simulink model "cubesat_alg_dev_env_v2_demoable"  (R2023a)
settings: Solver=FixedStepAuto  StartTime=0.0  StopTime=7200  FixedStep=0.01  MaxStep=1  MinStep=0.001  RelTol=1e-3
undefined symbols (not defined in the file or in its folder): WMM2020
libraries: aerolibutil x7, matrix_library x4, sharedtransform x2, dspinverses x1, sharedutil x1, simulink_extras x1, vrlib x1, aerolibgravity2 x1
settings Model: Creator=samuel  LastModifiedBy=samuel
settings OptimizationCC: ReuseModelBlockBuffer=off
settings ModelReferenceCC: EnableRefExpFcnMdlSchedulingChecks=on

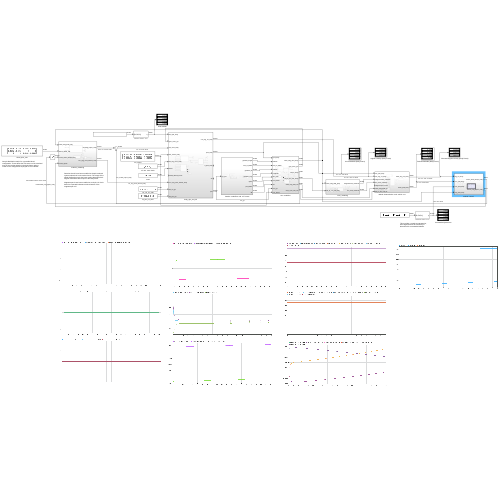
[thumbnail: Simulink's stored preview of the top-level diagram]
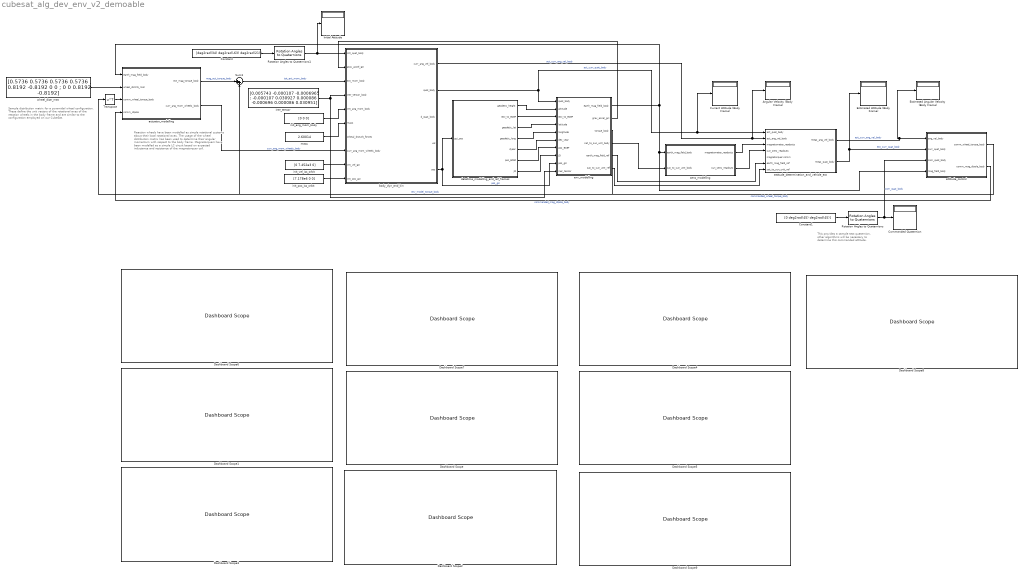
== system cubesat_alg_dev_env_v2_demoable ==
  note: This provides a sample test quaternion, other algorithms will be necessary to determine this commanded attitude.
  note: Reaction wheels have been modelled as simple rotational systems about their local rotational axes. The usage of the wheel distribution matrix has been used to determine their angular momentum with respect to the body frame.
      |
      | Magnetorquers have been modelled as a simple LC circuit based on expected inductance and resistance of the magnetorquer coil.
  note: Sample distribution matrix for a pyramidal wheel configuration. These define the unit vectors of the rotational axes of the reaction wheels in the body frame and are similar to the configuration employed on our CubeSat.
  Angular Velocity (Body Frame) : Display
  Commanded Quaternion : Display
  Constant : Constant  Value=[deg2rad(34) deg2rad(-63) deg2rad(21)]
  Constant1 : Constant  Value=[0 deg2rad(45) deg2rad(45)]
  Current Attitude (Body Frame) : Display
  Dashboard Scope{,1..9} (10 alike) : DashboardScope
  Estimated Angular Velocity (Body Frame) : Display
  Estimated Attitude (Body Frame) : Display
  Initial Attitude : Display
  Rotation Angles to Quaternions : sharedtransform/Rotation Angles to Quaternions  rotationOrder=ZYX  aMode=aMode
  Rotation Angles to Quaternions1 : sharedtransform/Rotation Angles to Quaternions  rotationOrder=ZYX  aMode=aMode
  Sum3 : Sum  Inputs=|++
  Transpose : Math  Operator=transpose
  actuator_modelling : Subsystem
  attitude_control : Subsystem
  attitude_determination_and_vehicle_est : Subsystem
  body_dyn_and_kin : Subsystem
  datetime_modelling_and_ref_frames : Subsystem
  env_modelling : Subsystem
  iner_tensor : Constant  Value=[0.005743 -0.000107 -0.0006965 ; -0.000107 0.030927 0.000086 ; -0.000696 0.000086 0.030951]
  init_ang_mom_body : Constant  Value=[0 0 0]
  init_pos_iss_orbit : Constant  Value=[7.178e6 0 0]
  init_vel_iss_orbit : Constant  Value=[0 7.452e3 0]
  mass : Constant  Value=2.60014
  sens_modelling : Subsystem
  wheel_distr_mat : Constant  Value=[0.5736 0.5736 0.5736 0.5736 ; 0.8192 -0.8192 0 0 ; 0 0 0.8192 -0.8192]
  wires:
  iner_tensor/1 -> env_modelling/10(iner_tensor), body_dyn_and_kin/4(iner_tensor_body)
  wheel_distr_mat/1 -> actuator_modelling/2(wheel_distrib_mat)
  actuator_modelling/1(ext_mag_torque_body) -> Sum3/1  "mag_act_torque_body"
  body_dyn_and_kin/2(quat_body) -> attitude_determination_and_vehicle_est/1(act_quat_body), Current Attitude (Body Frame)/1, env_modelling/1(quat_body)  "act_curr_quat_body"
  body_dyn_and_kin/5(pos) -> env_modelling/9(pos_gci), datetime_modelling_and_ref_frames/1(gci_pos)  "pos_gci"
  Sum3/1 -> body_dyn_and_kin/3(ext_mom_body)  "tot_ext_mom_body"
  init_ang_mom_body/1 -> body_dyn_and_kin/5(init_ang_mom_body)
  mass/1 -> body_dyn_and_kin/6(mass)
  actuator_modelling/2(curr_ang_mom_wheels_body) -> body_dyn_and_kin/8(curr_ang_mom_wheels_body)  "curr_ang_mom_wheels_body"
  init_vel_iss_orbit/1 -> body_dyn_and_kin/9(init_vel_gci)
  init_pos_iss_orbit/1 -> body_dyn_and_kin/10(init_pos_gci)
  env_modelling/1(earth_mag_field_body) -> attitude_control/4(mag_field_body), sens_modelling/1(earth_mag_field_body), actuator_modelling/1(earth_mag_field_body)
  datetime_modelling_and_ref_frames/1(geodetic_height) -> env_modelling/2(altitude)
  datetime_modelling_and_ref_frames/2(GCI_to_ECEF) -> env_modelling/3(GCI_to_ECEF)
  datetime_modelling_and_ref_frames/3(geodetic_lat) -> env_modelling/4(latitude)
  datetime_modelling_and_ref_frames/4(geodetic_long) -> env_modelling/5(longitude)
  datetime_modelling_and_ref_frames/5(dyear) -> env_modelling/6(dec_year)
  datetime_modelling_and_ref_frames/6(pos_ECEF) -> env_modelling/7(pos_ECEF)
  datetime_modelling_and_ref_frames/7(JD) -> env_modelling/8(JD)
  env_modelling/2(grav_accel_gci) -> body_dyn_and_kin/2(grav_accel_gci)
  env_modelling/3(torque_body) -> Sum3/2  "env_model_torque_body"
  env_modelling/4(sat_to_sun_unit_body) -> sens_modelling/2(sat_to_sun_unit_body)
  attitude_determination_and_vehicle_est/1(meas_ang_vel_body) -> Estimated Angular Velocity (Body Frame)/1, attitude_control/1(ang_vel_body)  "est_curr_ang_vel_body"
  attitude_determination_and_vehicle_est/2(meas_quat_body) -> Estimated Attitude (Body Frame)/1, attitude_control/2(curr_quat_body)  "est_curr_quat_body"
  attitude_control/1(comm_wheel_torque_body) -> Transpose/1  "commanded_wheel_torque_body"
  body_dyn_and_kin/1(curr_ang_vel_body) -> Angular Velocity (Body Frame)/1, attitude_determination_and_vehicle_est/2(act_ang_vel_body)  "act_curr_ang_vel_body"
  sens_modelling/1(magnetometer_readouts) -> attitude_determination_and_vehicle_est/3(magnetometer_readouts)
  sens_modelling/2(sun_sens_readouts) -> attitude_determination_and_vehicle_est/4(sun_sens_readouts)
  env_modelling/5(earth_mag_field_ref) -> attitude_determination_and_vehicle_est/6(earth_mag_field_ref)
  env_modelling/6(sat_to_sun_unit_ref) -> attitude_determination_and_vehicle_est/7(sat_to_sun_unit_ref)
  Transpose/1 -> actuator_modelling/3(comm_wheel_torque_body)
  Constant1/1 -> Rotation Angles to Quaternions/1
  Rotation Angles to Quaternions/1 -> Commanded Quaternion/1, attitude_control/3(com_quat_body)  "com_quat_body"
  Rotation Angles to Quaternions1/1 -> body_dyn_and_kin/1(init_quat_body), Initial Attitude/1
  Constant/1 -> Rotation Angles to Quaternions1/1
  attitude_control/2(comm_mag_dipole_body) -> actuator_modelling/4(comm_dipole)  "commanded_mag_dipole_body"

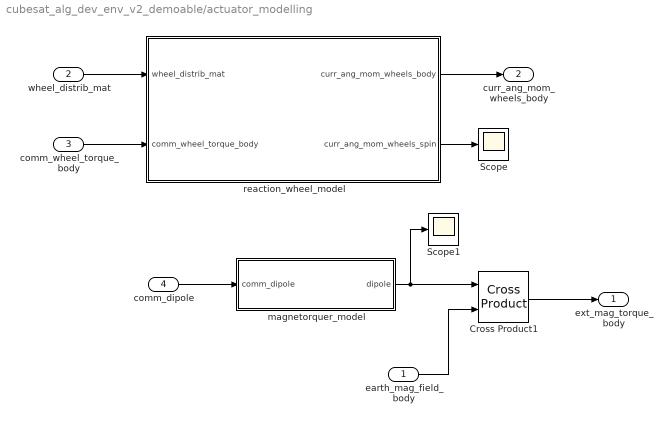
== system cubesat_alg_dev_env_v2_demoable/actuator_modelling ==
  earth_mag_field_body : Inport
  wheel_distrib_mat : Inport  Port=2
  comm_wheel_torque_body : Inport  Port=3
  comm_dipole : Inport  Port=4
  Cross Product1 : matrix_library/Cross Product
  Scope : Scope
  Scope1 : Scope
  magnetorquer_model : Subsystem
  reaction_wheel_model : Subsystem
  ext_mag_torque_body : Outport
  curr_ang_mom_wheels_body : Outport  Port=2
  wires:
  reaction_wheel_model/2(curr_ang_mom_wheels_spin) -> Scope/1
  magnetorquer_model/1(dipole) -> Scope1/1, Cross Product1/1
  Cross Product1/1 -> ext_mag_torque_body/1
  wheel_distrib_mat/1 -> reaction_wheel_model/1(wheel_distrib_mat)
  comm_wheel_torque_body/1 -> reaction_wheel_model/2(comm_wheel_torque_body)
  earth_mag_field_body/1 -> Cross Product1/2
  comm_dipole/1 -> magnetorquer_model/1(comm_dipole)
  reaction_wheel_model/1(curr_ang_mom_wheels_body) -> curr_ang_mom_wheels_body/1

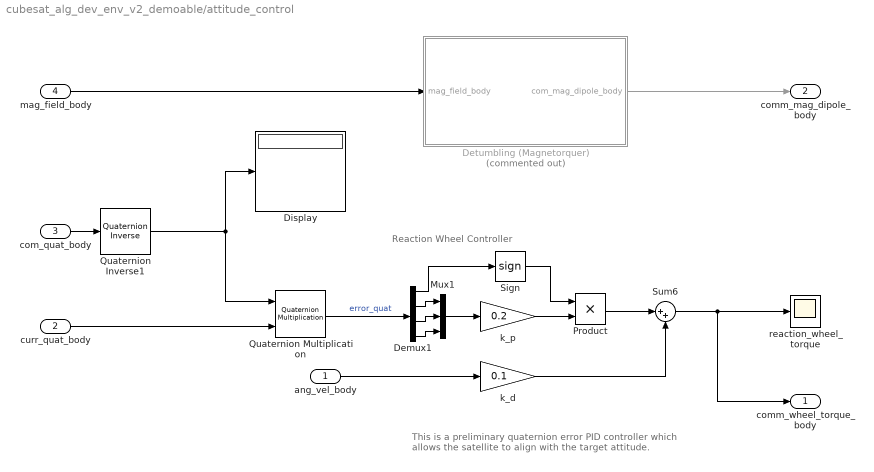
== system cubesat_alg_dev_env_v2_demoable/attitude_control ==
  note: This is a preliminary quaternion error PID controller which allows the satellite to align with the target attitude.
  note: Reaction Wheel Controller
  ang_vel_body : Inport
  curr_quat_body : Inport  Port=2
  com_quat_body : Inport  Port=3
  mag_field_body : Inport  Port=4
  Demux1 : Demux
  Detumbling (Magnetorquer) : Subsystem  Commented=on
  Display : Display
  Mux1 : Mux  Inputs=3
  Product : Product
  Quaternion Inverse1 : aerolibutil/Quaternion Inverse
  Quaternion Multiplication : aerolibutil/Quaternion Multiplication
  Sign : Signum
  Sum6 : Sum  Inputs=|++
  k_d : Gain  Gain=0.1
  k_p : Gain  Gain=0.2
  reaction_wheel_torque : Scope
  comm_wheel_torque_body : Outport
  comm_mag_dipole_body : Outport  Port=2
  wires:
  Quaternion Multiplication/1 -> Demux1/1  "error_quat"
  curr_quat_body/1 -> Quaternion Multiplication/2
  ang_vel_body/1 -> k_d/1
  Quaternion Inverse1/1 -> Display/1, Quaternion Multiplication/1
  Sum6/1 -> comm_wheel_torque_body/1, reaction_wheel_torque/1
  Demux1/3 -> Mux1/2
  Demux1/2 -> Mux1/1
  Demux1/4 -> Mux1/3
  k_p/1 -> Product/2
  Demux1/1 -> Sign/1
  Mux1/1 -> k_p/1
  Sign/1 -> Product/1
  Product/1 -> Sum6/1
  k_d/1 -> Sum6/2
  com_quat_body/1 -> Quaternion Inverse1/1
  mag_field_body/1 -> Detumbling (Magnetorquer)/1(mag_field_body)
  Detumbling (Magnetorquer)/1(com_mag_dipole_body) -> comm_mag_dipole_body/1

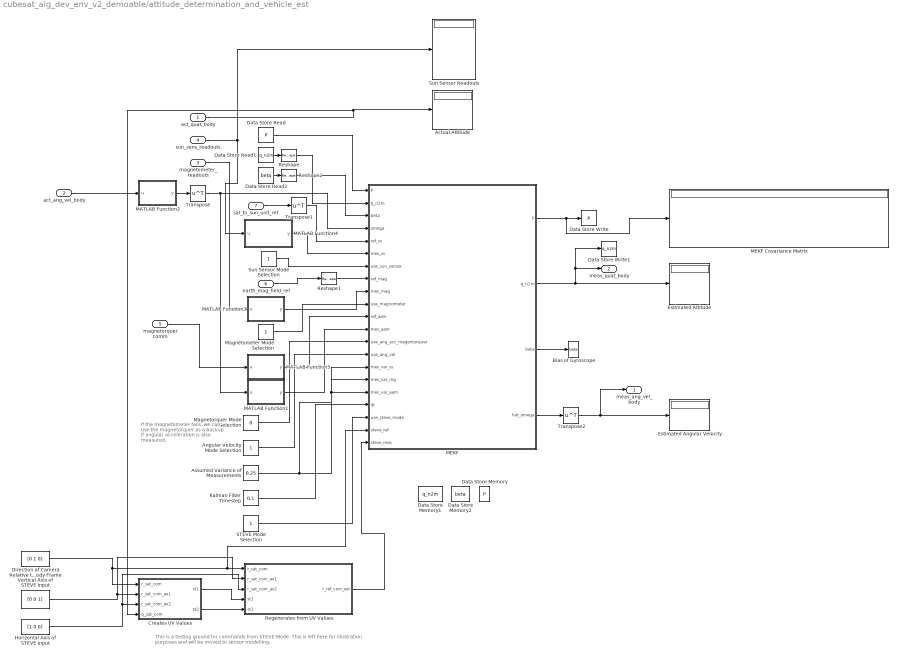
== system cubesat_alg_dev_env_v2_demoable/attitude_determination_and_vehicle_est ==
  note: This is a testing ground for commands from STEVE Mode. This is left here for illustration purposes and will be moved to sensor modelling.
  note: If the magnetometer fails, we can use the magnetorquer as a backup if angular acceleration is also measured.
  act_quat_body : Inport
  act_ang_vel_body : Inport  Port=2
  magnetometer_readouts : Inport  Port=3
  sun_sens_readouts : Inport  Port=4
  magnetorquer comm : Inport  Port=5
  earth_mag_field_ref : Inport  Port=6
  sat_to_sun_unit_ref : Inport  Port=7
  Actual Attitude : Display
  Angular Velocity Mode Selection : Constant
  Assumed Variance of Measurements : Constant  Value=0.25
  Bias of Gyroscope : DataStoreWrite  DataStoreName=beta  IndexOptions=Index vector (dialog)  Indices=1  OutputSizes=1
  Creates UV Values : MATLAB Function  TreatAsAtomicUnit=on
  Data Store Memory : DataStoreMemory  DataStoreName=P  WriteAfterWriteMsg=warning  InitialValue=diag([1*ones(1,3), 1*ones(1,3)])  ShowAdditionalParam=off
  Data Store Memory1 : DataStoreMemory  DataStoreName=q_n2m  WriteAfterWriteMsg=warning  InitialValue=[1, 0, 0, 0]  ShowAdditionalParam=off  Dimensions=[1,4]
  Data Store Memory2 : DataStoreMemory  DataStoreName=beta  WriteAfterWriteMsg=warning  InitialValue=[0;0;0]  ShowAdditionalParam=off  Dimensions=[3,1]
  Data Store Read : DataStoreRead  DataStoreName=P  IndexOptions=Index vector (dialog)  Indices=1  OutputSizes=1
  Data Store Read1 : DataStoreRead  DataStoreName=q_n2m  IndexOptions=Index vector (dialog)  Indices=1  OutputSizes=1
  Data Store Read2 : DataStoreRead  DataStoreName=beta  IndexOptions=Index vector (dialog)  Indices=1  OutputSizes=1
  Data Store Write : DataStoreWrite  DataStoreName=P  IndexOptions=Index vector (dialog)  Indices=1  OutputSizes=1
  Data Store Write1 : DataStoreWrite  DataStoreName=q_n2m  IndexOptions=Index vector (dialog)  Indices=1  OutputSizes=1
  Direction of Camera Relative to Body Frame : Constant  Value=[0 1 0]
  Estimated Angular Velocity : Display
  Estimated Attitude : Display
  Horizontal Axis of STEVE Input : Constant  Value=[1 0 0]
  Kalman Filter Timestep : Constant  Value=0.1
  MATLAB Function1 : MATLAB Function  TreatAsAtomicUnit=on
  MATLAB Function2 : MATLAB Function  TreatAsAtomicUnit=on
  MATLAB Function3 : MATLAB Function  TreatAsAtomicUnit=on
  MATLAB Function4 : MATLAB Function  TreatAsAtomicUnit=on
  MATLAB Function5 : MATLAB Function  TreatAsAtomicUnit=on
  MEKF : MATLAB Function  TreatAsAtomicUnit=on
  MEKF Covariance Matrix : Display
  Magnetometer Mode Selection : Constant
  Magnetorquer Mode Selection : Constant  Value=0
  Regenerates from UV Values : MATLAB Function  TreatAsAtomicUnit=on
  Reshape : Reshape  OutputDimensionality=Row vector (2-D)
  Reshape1 : Reshape  OutputDimensionality=Row vector (2-D)
  Reshape2 : Reshape  OutputDimensionality=Column vector (2-D)
  STEVE Mode Selection : Constant
  Sun Sensor Mode Selection : Constant
  Sun Sensor Readouts : Display
  Transpose : Math  Operator=transpose
  Transpose1 : Math  Operator=transpose
  Transpose2 : Math  Operator=transpose
  Vertical Axis of STEVE Input : Constant  Value=[0 0 1]
  meas_ang_vel_body : Outport
  meas_quat_body : Outport  Port=2
  wires:
  MEKF/3(beta) -> Bias of Gyroscope/1
  MEKF/2(q_n2m) -> Data Store Write1/1, meas_quat_body/1, Estimated Attitude/1
  Magnetometer Mode Selection/1 -> MEKF/10(use_magnometer)
  Magnetorquer Mode Selection/1 -> MEKF/13(use_ang_acc_magentorquer)
  sun_sens_readouts/1 -> Sun Sensor Readouts/1, MATLAB Function4/1(u)
  Angular Velocity Mode Selection/1 -> MEKF/14(use_ang_vel)
  MATLAB Function2/1(y) -> Transpose/1
  MEKF/4(hat_omega) -> Transpose2/1
  Data Store Read/1 -> MEKF/1("P ")
  MATLAB Function1/1(y) -> MEKF/12(mes_aam)
  earth_mag_field_ref/1 -> Reshape1/1
  act_ang_vel_body/1 -> MATLAB Function2/1(u)
  Data Store Read2/1 -> Reshape2/1
  sat_to_sun_unit_ref/1 -> Transpose1/1
  magnetometer_readouts/1 -> MATLAB Function3/1(u)
  MATLAB Function5/1(y) -> MEKF/11(ref_aam)
  magnetorquer comm/1 -> MATLAB Function5/1(u)
  Sun Sensor Mode Selection/1 -> MEKF/7(use_sun_sensor)
  MATLAB Function3/1(y) -> MEKF/9(mes_mag)
  Assumed Variance of Measurements/1 -> MEKF/17(mes_var_aam), MEKF/16(mes_var_mg), MEKF/15(mes_var_ss)
  Kalman Filter Timestep/1 -> MEKF/18(dt)
  Transpose/1 -> MATLAB Function1/1(u), MEKF/4(omega)
  Transpose1/1 -> MEKF/5(ref_ss)
  Reshape1/1 -> MEKF/8(ref_mag)
  Data Store Read1/1 -> Reshape/1
  Reshape2/1 -> MEKF/3("beta ")
  Transpose2/1 -> meas_ang_vel_body/1, Estimated Angular Velocity/1
  MEKF/1(P) -> MEKF Covariance Matrix/1, Data Store Write/1
  Reshape/1 -> MEKF/2("q_n2m ")
  act_quat_body/1 -> Creates UV Values/4(q_sat_com), Actual Attitude/1
  MATLAB Function4/1(y) -> MEKF/6(mes_ss)
  Creates UV Values/1(st1) -> Regenerates from UV Values/4(st1)
  Creates UV Values/2(st2) -> Regenerates from UV Values/5(st2)
  Horizontal Axis of STEVE Input/1 -> Regenerates from UV Values/3(r_sat_com_ax2), Creates UV Values/3(r_sat_com_ax2)
  Vertical Axis of STEVE Input/1 -> Regenerates from UV Values/2(r_sat_com_ax1), Creates UV Values/2(r_sat_com_ax1)
  Direction of Camera Relative to Body Frame/1 -> Creates UV Values/1(r_sat_com), MEKF/20(steve_ref), Regenerates from UV Values/1(r_sat_com)
  Regenerates from UV Values/1(r_ref_com_est) -> MEKF/21(steve_mes)
  STEVE Mode Selection/1 -> MEKF/19(use_steve_mode)

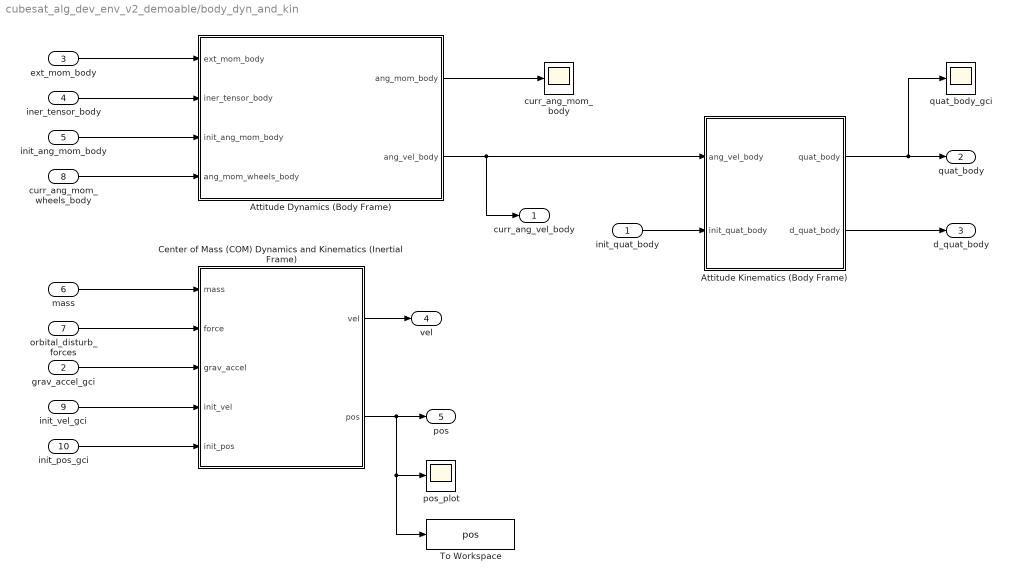
== system cubesat_alg_dev_env_v2_demoable/body_dyn_and_kin ==
  init_quat_body : Inport
  grav_accel_gci : Inport  Port=2
  ext_mom_body : Inport  Port=3
  iner_tensor_body : Inport  Port=4
  init_ang_mom_body : Inport  Port=5
  mass : Inport  Port=6
  orbital_disturb_forces : Inport  Port=7
  curr_ang_mom_wheels_body : Inport  Port=8
  init_vel_gci : Inport  Port=9
  init_pos_gci : Inport  Port=10
  Attitude Dynamics (Body Frame) : Subsystem
  Attitude Kinematics (Body Frame) : Subsystem
  Center of Mass (COM) Dynamics and Kinematics (Inertial Frame) : Subsystem
  To Workspace : ToWorkspace  VariableName=pos  SampleTime=-1
  curr_ang_mom_body : Scope
  pos_plot : Scope
  quat_body_gci : Scope
  curr_ang_vel_body : Outport
  quat_body : Outport  Port=2
  d_quat_body : Outport  Port=3
  vel : Outport  Port=4
  pos : Outport  Port=5
  wires:
  init_quat_body/1 -> Attitude Kinematics (Body Frame)/2(init_quat_body)
  grav_accel_gci/1 -> Center of Mass (COM) Dynamics and Kinematics (Inertial Frame)/3(grav_accel)
  ext_mom_body/1 -> Attitude Dynamics (Body Frame)/1(ext_mom_body)
  Attitude Dynamics (Body Frame)/2(ang_vel_body) -> Attitude Kinematics (Body Frame)/1(ang_vel_body), curr_ang_vel_body/1
  iner_tensor_body/1 -> Attitude Dynamics (Body Frame)/2(iner_tensor_body)
  init_vel_gci/1 -> Center of Mass (COM) Dynamics and Kinematics (Inertial Frame)/4(init_vel)
  orbital_disturb_forces/1 -> Center of Mass (COM) Dynamics and Kinematics (Inertial Frame)/2(force)
  curr_ang_mom_wheels_body/1 -> Attitude Dynamics (Body Frame)/4(ang_mom_wheels_body)
  init_pos_gci/1 -> Center of Mass (COM) Dynamics and Kinematics (Inertial Frame)/5(init_pos)
  Center of Mass (COM) Dynamics and Kinematics (Inertial Frame)/2(pos) -> To Workspace/1, pos_plot/1, pos/1
  Attitude Kinematics (Body Frame)/2(d_quat_body) -> d_quat_body/1
  Attitude Kinematics (Body Frame)/1(quat_body) -> quat_body_gci/1, quat_body/1
  mass/1 -> Center of Mass (COM) Dynamics and Kinematics (Inertial Frame)/1(mass)
  init_ang_mom_body/1 -> Attitude Dynamics (Body Frame)/3(init_ang_mom_body)
  Attitude Dynamics (Body Frame)/1(ang_mom_body) -> curr_ang_mom_body/1
  Center of Mass (COM) Dynamics and Kinematics (Inertial Frame)/1(vel) -> vel/1

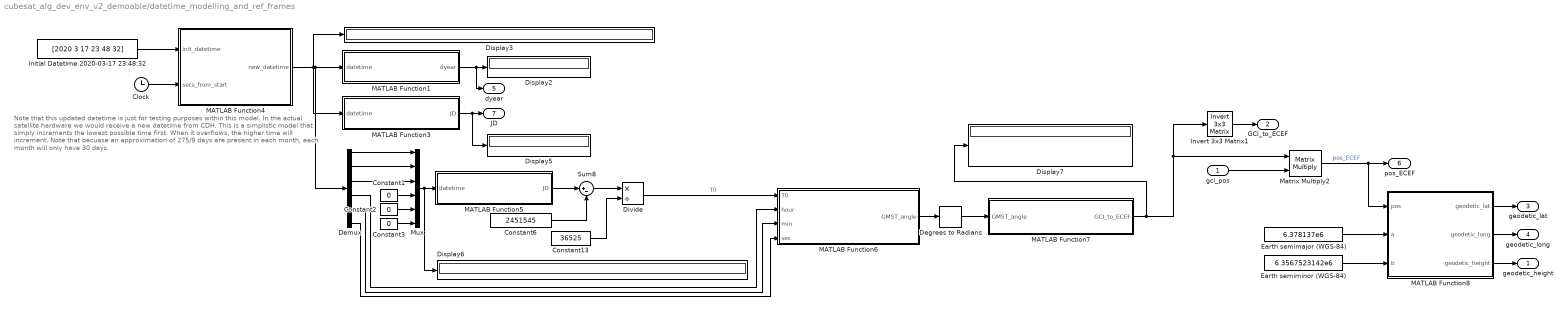
== system cubesat_alg_dev_env_v2_demoable/datetime_modelling_and_ref_frames ==
  note: Note that this updated datetime is just for testing purposes within this model. In the actual satellite hardware we would receive a new datetime from CDH. This is a simplistic model that simply increments the lowest possible time first. When it overflows, the higher time will increment. Note that becuase an approximation of 275/9 days are present in each month, each month will only have 30 days.
  gci_pos : Inport
  Clock : Clock
  Constant1 : Constant  Value=0
  Constant13 : Constant  Value=36525
  Constant2 : Constant  Value=0
  Constant3 : Constant  Value=0
  Constant6 : Constant  Value=2451545
  Degrees to Radians : simulink_extras/Transformations/Degrees to Radians
  Demux : Demux  Outputs=6
  Display{2..3,5..7} (5 alike) : Display
  Divide : Product  Inputs=*/
  Earth semimajor (WGS-84) : Constant  Value=6.378137e6
  Earth semiminor (WGS-84) : Constant  Value=6.3567523142e6
  Initial Datetime 2020-03-17 23:48:32 : Constant  Value=[2020 3 17 23 48 32]
  Invert 3x3 Matrix1 : aerolibutil/Invert  3x3 Matrix
  MATLAB Function1 : MATLAB Function  TreatAsAtomicUnit=on
  MATLAB Function3 : MATLAB Function  TreatAsAtomicUnit=on
  MATLAB Function4 : MATLAB Function  TreatAsAtomicUnit=on
  MATLAB Function5 : MATLAB Function  TreatAsAtomicUnit=on
  MATLAB Function6 : MATLAB Function  TreatAsAtomicUnit=on
  MATLAB Function7 : MATLAB Function  TreatAsAtomicUnit=on
  MATLAB Function8 : MATLAB Function  TreatAsAtomicUnit=on
  Matrix Multiply2 : Product  Multiplication=Matrix(*)
  Mux : Mux  Inputs=6
  Sum8 : Sum  Inputs=|+-
  geodetic_height : Outport
  GCI_to_ECEF : Outport  Port=2
  geodetic_lat : Outport  Port=3
  geodetic_long : Outport  Port=4
  dyear : Outport  Port=5
  pos_ECEF : Outport  Port=6
  JD : Outport  Port=7
  wires:
  Constant3/1 -> Mux/6
  MATLAB Function8/1(geodetic_lat) -> geodetic_lat/1
  Divide/1 -> MATLAB Function6/1(T0)  "T0"
  MATLAB Function4/1(new_datetime) -> Demux/1, MATLAB Function1/1(datetime), MATLAB Function3/1(datetime), Display3/1
  MATLAB Function6/1(GMST_angle) -> Degrees to Radians/1
  MATLAB Function1/1(dyear) -> dyear/1, Display2/1
  Invert 3x3 Matrix1/1 -> GCI_to_ECEF/1
  MATLAB Function3/1(JD) -> Display5/1, JD/1
  MATLAB Function8/3(geodetic_height) -> geodetic_height/1
  MATLAB Function8/2(geodetic_long) -> geodetic_long/1
  Constant1/1 -> Mux/4
  Demux/5 -> MATLAB Function6/3(min)
  Demux/1 -> Mux/1
  Sum8/1 -> Divide/1
  Constant13/1 -> Divide/2
  Earth semiminor (WGS-84)/1 -> MATLAB Function8/3(b)
  Earth semimajor (WGS-84)/1 -> MATLAB Function8/2(a)
  Matrix Multiply2/1 -> MATLAB Function8/1(pos), pos_ECEF/1  "pos_ECEF"
  Demux/6 -> MATLAB Function6/4(sec)
  Constant6/1 -> Sum8/2
  gci_pos/1 -> Matrix Multiply2/2
  MATLAB Function5/1(JD) -> Sum8/1
  MATLAB Function7/1(GCI_to_ECEF) -> Matrix Multiply2/1, Invert 3x3 Matrix1/1, Display7/1
  Degrees to Radians/1 -> MATLAB Function7/1(GMST_angle)
  Mux/1 -> Display6/1, MATLAB Function5/1(datetime)
  Initial Datetime 2020-03-17 23:48:32/1 -> MATLAB Function4/1(init_datetime)
  Clock/1 -> MATLAB Function4/2(secs_from_start)
  Demux/3 -> Mux/3
  Demux/4 -> MATLAB Function6/2(hour)
  Demux/2 -> Mux/2
  Constant2/1 -> Mux/5

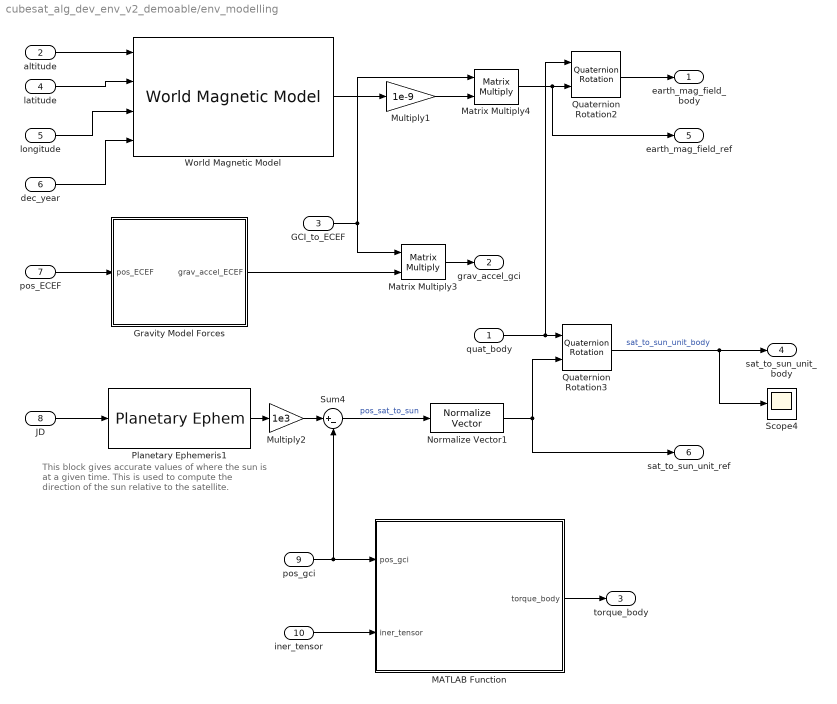
== system cubesat_alg_dev_env_v2_demoable/env_modelling ==
  note: This block gives accurate values of where the sun is at a given time. This is used to compute the direction of the sun relative to the satellite.
  quat_body : Inport
  altitude : Inport  Port=2
  GCI_to_ECEF : Inport  Port=3
  latitude : Inport  Port=4
  longitude : Inport  Port=5
  dec_year : Inport  Port=6
  pos_ECEF : Inport  Port=7
  JD : Inport  Port=8
  pos_gci : Inport  Port=9
  iner_tensor : Inport  Port=10
  Gravity Model Forces : Subsystem
  MATLAB Function : MATLAB Function  TreatAsAtomicUnit=on
  Matrix Multiply3 : Product  Multiplication=Matrix(*)
  Matrix Multiply4 : Product  Multiplication=Matrix(*)
  Multiply1 : Gain  Gain=1e-9
  Multiply2 : Gain  Gain=1e3
  Normalize Vector1 : vrlib/Utilities/Normalize Vector  maxzero=0
  Planetary Ephemeris1 : PlanetaryEphem  target=Sun  outputVelocity=off
  Quaternion Rotation2 : aerolibutil/Quaternion Rotation
  Quaternion Rotation3 : aerolibutil/Quaternion Rotation
  Scope4 : Scope
  Sum4 : Sum  Inputs=|+-
  World Magnetic Model : aerolibgravity2/World Magnetic Model  model=WMM2020 (2020-2025)  customFile='WMM2020.COF'  units=Metric (MKS)  time_in=on  month=January  day=1  year=2020  action=Error  h_out=off  dec_out=off  inc_out=off  ti_out=off
  earth_mag_field_body : Outport
  grav_accel_gci : Outport  Port=2
  torque_body : Outport  Port=3
  sat_to_sun_unit_body : Outport  Port=4
  earth_mag_field_ref : Outport  Port=5
  sat_to_sun_unit_ref : Outport  Port=6
  wires:
  Normalize Vector1/1 -> sat_to_sun_unit_ref/1, Quaternion Rotation3/2
  Matrix Multiply4/1 -> earth_mag_field_ref/1, Quaternion Rotation2/2
  dec_year/1 -> World Magnetic Model/4
  MATLAB Function/1(torque_body) -> torque_body/1
  pos_ECEF/1 -> Gravity Model Forces/1(pos_ECEF)
  World Magnetic Model/1 -> Multiply1/1
  Planetary Ephemeris1/1 -> Multiply2/1
  Matrix Multiply3/1 -> grav_accel_gci/1
  Multiply2/1 -> Sum4/1
  Quaternion Rotation3/1 -> Scope4/1, sat_to_sun_unit_body/1  "sat_to_sun_unit_body"
  altitude/1 -> World Magnetic Model/1
  JD/1 -> Planetary Ephemeris1/1
  pos_gci/1 -> MATLAB Function/1(pos_gci), Sum4/2
  Gravity Model Forces/1(grav_accel_ECEF) -> Matrix Multiply3/2
  longitude/1 -> World Magnetic Model/3
  GCI_to_ECEF/1 -> Matrix Multiply4/1, Matrix Multiply3/1
  Multiply1/1 -> Matrix Multiply4/2
  latitude/1 -> World Magnetic Model/2
  iner_tensor/1 -> MATLAB Function/2(iner_tensor)
  quat_body/1 -> Quaternion Rotation3/1, Quaternion Rotation2/1
  Quaternion Rotation2/1 -> earth_mag_field_body/1
  Sum4/1 -> Normalize Vector1/1  "pos_sat_to_sun"

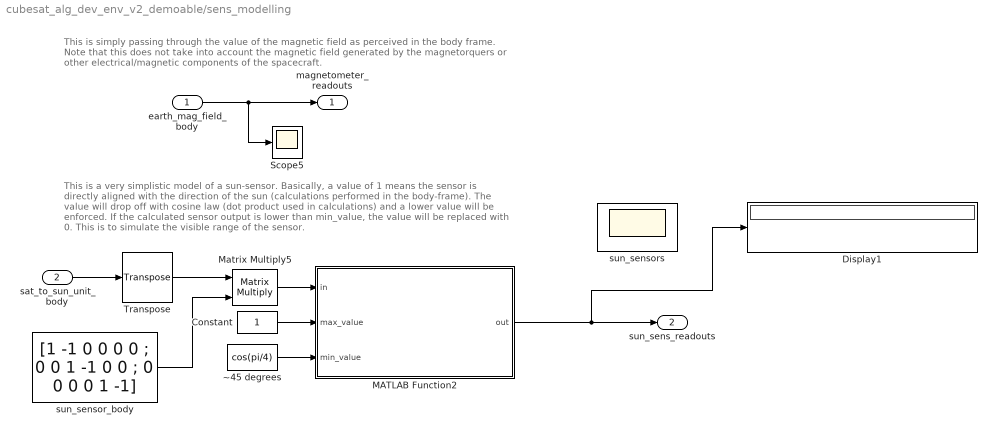
== system cubesat_alg_dev_env_v2_demoable/sens_modelling ==
  note: This is simply passing through the value of the magnetic field as perceived in the body frame. Note that this does not take into account the magnetic field generated by the magnetorquers or other electrical/magnetic components of the spacecraft.
  note: This is a very simplistic model of a sun-sensor. Basically, a value of 1 means the sensor is directly aligned with the direction of the sun (calculations performed in the body-frame). The value will drop off with cosine law (dot product used in calculations) and a lower value will be enforced. If the calculated sensor output is lower than min_value, the value will be replaced with 0. This is to simulate the visible range of the sensor.
  earth_mag_field_body : Inport
  sat_to_sun_unit_body : Inport  Port=2
  Constant : Constant
  Display1 : Display
  MATLAB Function2 : MATLAB Function  TreatAsAtomicUnit=on
  Matrix Multiply5 : Product  Multiplication=Matrix(*)
  Scope5 : Scope
  Transpose : matrix_library/Transpose
  sun_sensor_body : Constant  Value=[1 -1 0 0 0 0 ; 0 0 1 -1 0 0 ; 0 0 0 0 1 -1]
  sun_sensors : Scope
  ~45 degrees : Constant  Value=cos(pi/4)
  magnetometer_readouts : Outport
  sun_sens_readouts : Outport  Port=2
  wires:
  sun_sensor_body/1 -> Matrix Multiply5/2
  ~45 degrees/1 -> MATLAB Function2/3(min_value)
  Transpose/1 -> Matrix Multiply5/1
  Constant/1 -> MATLAB Function2/2(max_value)
  Matrix Multiply5/1 -> MATLAB Function2/1(in)
  earth_mag_field_body/1 -> Scope5/1, magnetometer_readouts/1
  sat_to_sun_unit_body/1 -> Transpose/1
  MATLAB Function2/1(out) -> Display1/1, sun_sens_readouts/1

== system cubesat_alg_dev_env_v2_demoable/actuator_modelling/magnetorquer_model ==
  comm_dipole : Inport
  Demux : Demux  Outputs=3
  Mux : Mux  Inputs=3
  State-Space : StateSpace  A=-71.31  B=8  C=8.914  D=0  InitialCondition=0
  State-Space1 : StateSpace  A=-71.31  B=8  C=8.914  D=0  InitialCondition=0
  State-Space2 : StateSpace  A=-71.31  B=8  C=8.914  D=0  InitialCondition=0
  dipole : Outport
  wires:
  State-Space/1 -> Mux/1
  State-Space2/1 -> Mux/3
  State-Space1/1 -> Mux/2
  Demux/2 -> State-Space1/1
  Demux/1 -> State-Space/1
  Demux/3 -> State-Space2/1
  Mux/1 -> dipole/1
  comm_dipole/1 -> Demux/1

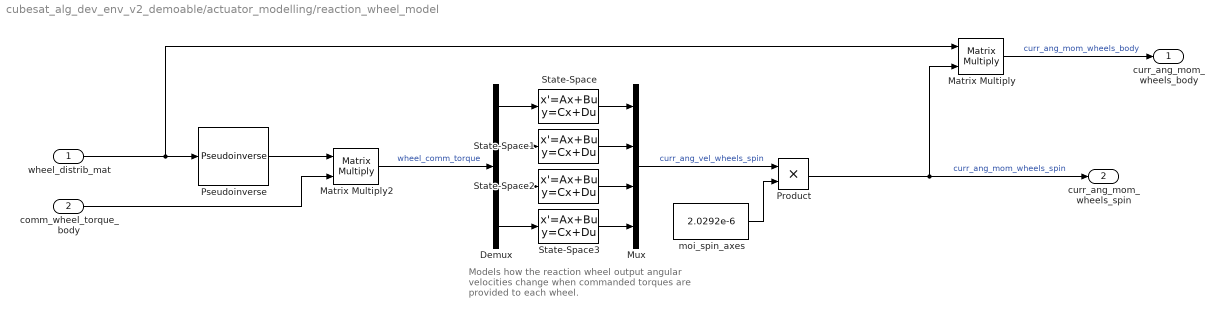
== system cubesat_alg_dev_env_v2_demoable/actuator_modelling/reaction_wheel_model ==
  note: Models how the reaction wheel output angular velocities change when commanded torques are provided to each wheel.
  wheel_distrib_mat : Inport
  comm_wheel_torque_body : Inport  Port=2
  Demux : Demux
  Matrix Multiply : Product  Multiplication=Matrix(*)
  Matrix Multiply2 : Product  Multiplication=Matrix(*)
  Mux : Mux
  Product : Product
  Pseudoinverse : dspinverses/Pseudoinverse  wanterr=off  SimulateUsing=Interpreted execution
  State-Space{,1..3} (4 alike) : StateSpace  A=-0.02216  B=512  C=962.5  D=0  InitialCondition=0  ParameterTunability=Unconstrained
  moi_spin_axes : Constant  Value=2.0292e-6
  curr_ang_mom_wheels_body : Outport
  curr_ang_mom_wheels_spin : Outport  Port=2
  wires:
  Demux/1 -> State-Space/1
  Demux/2 -> State-Space1/1
  Demux/4 -> State-Space3/1
  State-Space/1 -> Mux/1
  Pseudoinverse/1 -> Matrix Multiply2/1
  wheel_distrib_mat/1 -> Matrix Multiply/1, Pseudoinverse/1
  State-Space1/1 -> Mux/2
  moi_spin_axes/1 -> Product/2
  Mux/1 -> Product/1  "curr_ang_vel_wheels_spin"
  Product/1 -> curr_ang_mom_wheels_spin/1, Matrix Multiply/2  "curr_ang_mom_wheels_spin"
  Matrix Multiply2/1 -> Demux/1  "wheel_comm_torque"
  State-Space3/1 -> Mux/4
  State-Space2/1 -> Mux/3
  Demux/3 -> State-Space2/1
  comm_wheel_torque_body/1 -> Matrix Multiply2/2
  Matrix Multiply/1 -> curr_ang_mom_wheels_body/1  "curr_ang_mom_wheels_body"

== system cubesat_alg_dev_env_v2_demoable/attitude_control/Detumbling (Magnetorquer) ==
  note: This works for initial detumbling (control law approximation prior to getting attitude estimates)!! Note reaction wheel control laws disabled (other magnetorquer control law will be needed for momentum dumping but we have formula).
  mag_field_body : Inport
  Calculates magntiude of magnetic field : Sqrt
  Derivative : Derivative
  Divide : Product  Inputs=*/
  Dot Product : DotProduct  OutDataTypeStr=Inherit: Inherit via internal rule
  Gain : Gain  Gain=-1000
  Scope6 : Scope
  com_mag_dipole_body : Outport
  wires:
  Calculates magntiude of magnetic field/1 -> Divide/2
  Gain/1 -> com_mag_dipole_body/1
  Dot Product/1 -> Calculates magntiude of magnetic field/1
  Divide/1 -> Gain/1
  mag_field_body/1 -> Derivative/1, Dot Product/2, Dot Product/1
  Derivative/1 -> Divide/1, Scope6/1

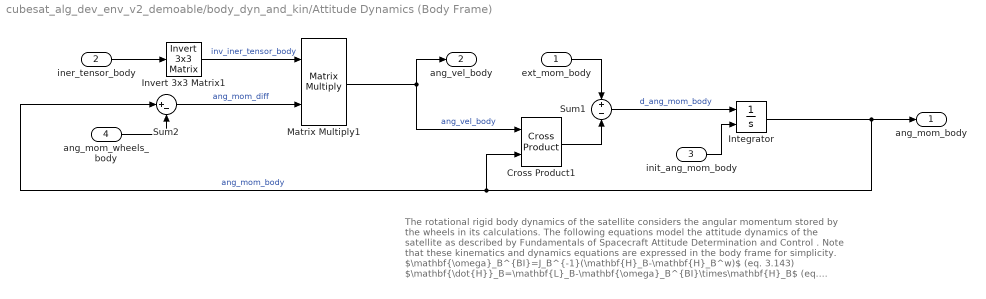
== system cubesat_alg_dev_env_v2_demoable/body_dyn_and_kin/Attitude Dynamics (Body Frame) ==
  note: The rotational rigid body dynamics of the satellite considers the angular momentum stored by the wheels in its calculations. The following equations model the attitude dynamics of the satellite as described by Fundamentals of Spacecraft Attitude Determination and Control . Note that these kinematics and dynamics equations are expressed in the body frame for simplicity.
      |
      | $\mathbf{\omega}_B^{BI}=J_B^{-1}(\mathbf{H}_B-\mathbf{H}_B^w)$ (eq. 3.143)
      | $\mathbf{\dot{H}}_B=\mathbf{L}_B-\mathbf{\omega}_B^{BI}\times\mathbf{H}_B$ (eq. 3.80)
      |
      | $\mathbf{\omega}_B^{BI}$ - angular velocity of satellite in body frame
      | $J_B$ - inertia tensor of satellite in body frame
      | $\mathbf{H}_B$ - total angular momentum of satellite in body frame
      | $\mathbf{H}_B^w$ - total angular momentum of wheels in body frame
      | $\mathbf{L}_B$ - moment applied to spacecraft in the body frame
  ext_mom_body : Inport
  iner_tensor_body : Inport  Port=2
  init_ang_mom_body : Inport  Port=3
  ang_mom_wheels_body : Inport  Port=4
  Cross Product1 : matrix_library/Cross Product
  Integrator : Integrator  InitialConditionSource=external
  Invert 3x3 Matrix1 : aerolibutil/Invert  3x3 Matrix
  Matrix Multiply1 : Product  Multiplication=Matrix(*)
  Sum1 : Sum  Inputs=+-
  Sum2 : Sum  Inputs=|+-
  ang_mom_body : Outport
  ang_vel_body : Outport  Port=2
  wires:
  Invert 3x3 Matrix1/1 -> Matrix Multiply1/1  "inv_iner_tensor_body"
  iner_tensor_body/1 -> Invert 3x3 Matrix1/1
  ang_mom_wheels_body/1 -> Sum2/2
  Integrator/1 -> ang_mom_body/1, Sum2/1, Cross Product1/2  "ang_mom_body"
  init_ang_mom_body/1 -> Integrator/2
  Matrix Multiply1/1 -> Cross Product1/1, ang_vel_body/1  "ang_vel_body"
  Sum2/1 -> Matrix Multiply1/2  "ang_mom_diff"
  Sum1/1 -> Integrator/1  "d_ang_mom_body"
  ext_mom_body/1 -> Sum1/1
  Cross Product1/1 -> Sum1/2

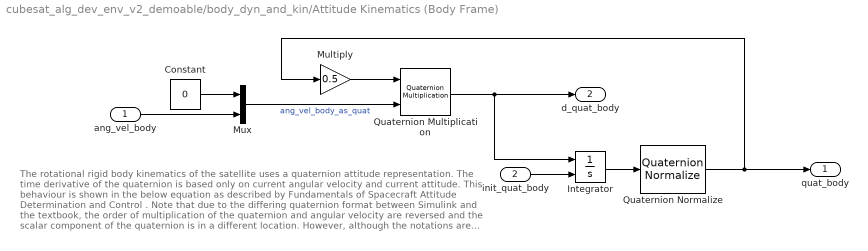
== system cubesat_alg_dev_env_v2_demoable/body_dyn_and_kin/Attitude Kinematics (Body Frame) ==
  note: The rotational rigid body kinematics of the satellite uses a quaternion attitude representation. The time derivative of the quaternion is based only on current angular velocity and current attitude. This behaviour is shown in the below equation as described by Fundamentals of Spacecraft Attitude Determination and Control . Note that due to the differing quaternion format between Simulink and the textbook, the order of multiplication of the quaternion and angular velocity are reversed and the scalar component of the quaternion is in a different location. However, although the notations are different, they are functionally the same.
      |
      | $\mathbf{\dot{q}}_{BI}=\frac{1}{2}\mathbf{q}_{BI}\cdot\mathbf{\omega}_B^{BI}=\frac{1}{2}\mathbf{q}_{BI}\cdot\left[\matrix{0 \cr \mathbf{\omega}_B^{BI}}\right]$ (eq. 3.79d)
      |
      | Note that in the above equation, multiplication between a quaternion and vector requires transforming the vector to a quaternion with scalar component of 0, as seen on the RHS.
      |
      | $\mathbf{q}_{BI}$ - current attitude of the spacecraft (rotation from inertial frame to body frame as specified in the inertial frame)
      | $\mathbf{\omega}_{B}^{BI}$ - angular velocity of satellite in body frame
  ang_vel_body : Inport
  init_quat_body : Inport  Port=2
  Constant : Constant  Value=0
  Integrator : Integrator  InitialConditionSource=external
  Multiply : Gain  Gain=0.5
  Mux : Mux  Inputs=2
  Quaternion Multiplication : aerolibutil/Quaternion Multiplication
  Quaternion Normalize : sharedutil/Quaternion Normalize  aMode=aMode
  quat_body : Outport
  d_quat_body : Outport  Port=2
  wires:
  Constant/1 -> Mux/1
  ang_vel_body/1 -> Mux/2
  Multiply/1 -> Quaternion Multiplication/1
  init_quat_body/1 -> Integrator/2
  Quaternion Multiplication/1 -> d_quat_body/1, Integrator/1
  Mux/1 -> Quaternion Multiplication/2  "ang_vel_body_as_quat"
  Integrator/1 -> Quaternion Normalize/1
  Quaternion Normalize/1 -> Multiply/1, quat_body/1

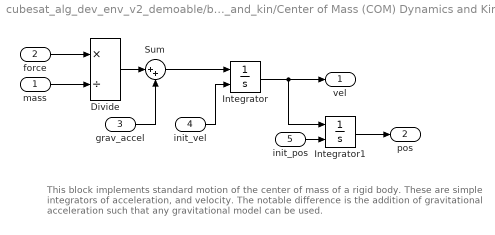
== system cubesat_alg_dev_env_v2_demoable/body_dyn_and_kin/Center of Mass (COM) Dynamics and Kinematics (Inertial Frame) ==
  note: This block implements standard motion of the center of mass of a rigid body. These are simple integrators of acceleration, and velocity. The notable difference is the addition of gravitational acceleration such that any gravitational model can be used.
  mass : Inport
  force : Inport  Port=2
  grav_accel : Inport  Port=3
  init_vel : Inport  Port=4
  init_pos : Inport  Port=5
  Divide : Product  Inputs=*/
  Integrator : Integrator  InitialConditionSource=external
  Integrator1 : Integrator  InitialConditionSource=external
  Sum : Sum  Inputs=|++
  vel : Outport
  pos : Outport  Port=2
  wires:
  init_vel/1 -> Integrator/2
  init_pos/1 -> Integrator1/2
  Divide/1 -> Sum/1
  grav_accel/1 -> Sum/2
  mass/1 -> Divide/2
  force/1 -> Divide/1
  Integrator/1 -> vel/1, Integrator1/1
  Integrator1/1 -> pos/1
  Sum/1 -> Integrator/1

== system cubesat_alg_dev_env_v2_demoable/env_modelling/Gravity Model Forces ==
  pos_ECEF : Inport
  Spherical Harmonic Gravity Model : SHGravity
  Transpose : matrix_library/Transpose
  grav_accel_ECEF : Outport
  wires:
  Spherical Harmonic Gravity Model/1 -> Transpose/1
  Transpose/1 -> grav_accel_ECEF/1
  pos_ECEF/1 -> Spherical Harmonic Gravity Model/1

== matlab function cubesat_alg_dev_env_v2_demoable/sens_modelling/MATLAB Function2 ==
  data: in input; out output; max_value input; min_value input
function out = zero_out_out_of_range(in, max_value, min_value)
    out = in;

    for i = 1:length(in)
        if out(i) < min_value || out(i) > max_value
            out(i) = 0;
        end
    end

== matlab function cubesat_alg_dev_env_v2_demoable/datetime_modelling_and_ref_frames/MATLAB Function3 ==
  data: datetime input; JD output
function JD = calc_JD_from_datetime(datetime)

% the datetime format is provided as a 6 value array
% year, month, day, hour, minute, second

% calculates the Julian date (JD) from the datetime
JD = 1721013.5 + 367*datetime(1) - floor(7/4*(datetime(1) + ...
    floor((datetime(2) + 9)/12))) + floor(275/9*datetime(2)) + ...
    datetime(3) + (60*datetime(4) + datetime(5) + datetime(6)/60)/1440;

% note that seconds should be /61 for leap days but since we are using a
% testing environment we do not need to worry about this

% presumably in the navigation system of the actual satellite we may also
% not need to consider this as it would introduce a negligible error or we
% may need to have some special protocol with CDH to figure out a system

== matlab function cubesat_alg_dev_env_v2_demoable/datetime_modelling_and_ref_frames/MATLAB Function4 ==
  data: init_datetime input; new_datetime output; secs_from_start input
function new_datetime  = datetime_upd(init_datetime, secs_from_start)

% the datetime format is provided as a 6 value array
% year, month, day, hour, minute, second

% initializes new datetime array
new_datetime = zeros(1, 6);

% adds the seconds from start of simulation to seconds
new_datetime(6) = init_datetime(6) + secs_from_start;

% computes the new seconds and minutes with carry over
new_datetime(5) = init_datetime(5) + floor(new_datetime(6) / 60);
new_datetime(6) = mod(new_datetime(6), 60);

% computes the new minutes and hours with carry over
new_datetime(4) = init_datetime(4) + floor(new_datetime(5) / 60);
new_datetime(5) = mod(new_datetime(5), 60);

% computes the new hours and days with carry over
new_datetime(3) = init_datetime(3) + floor(new_datetime(4) / 24);
new_datetime(4) = mod(new_datetime(4), 24);

% computes the new days and months with carry over
new_datetime(2) = init_datetime(2) + floor(new_datetime(3) / (275/9));

% NOTE: the floor here is specifically needed to prevent a recurring
% decimal from occurring here due to using an average number of days per
% month of 275/9 (this also caps days in a month to 30)
new_datetime(3) = floor(mod(new_datetime(3), (275/9)));

% computes the new months and years with carry over

% for calculations, shifts first month to 0
new_datetime(2) = new_datetime(2) - 1;

new_datetime(1) = init_datetime(1) + floor(new_datetime(2) / 12);

% done with calculations, restores first month to 1
new_datetime(2) = mod(new_datetime(2), 12) + 1;

end

== matlab function cubesat_alg_dev_env_v2_demoable/datetime_modelling_and_ref_frames/MATLAB Function5 ==
  data: datetime input; JD output
function JD = calc_JD_from_datetime(datetime)

% the datetime format is provided as a 6 value array
% year, month, day, hour, minute, second

% calculates the Julian date (JD) from the datetime
JD = 1721013.5 + 367*datetime(1) - floor(7/4*(datetime(1) + ...
    floor((datetime(2) + 9)/12))) + floor(275/9*datetime(2)) + ...
    datetime(3) + (60*datetime(4) + datetime(5) + datetime(6)/60)/1440;

% note that seconds should be /61 for leap days but since we are using a
% testing environment we do not need to worry about this

% presumably in the navigation system of the actual satellite we may also
% not need to consider this as it would introduce a negligible error or we
% may need to have some special protocol with CDH to figure out a system

== matlab function cubesat_alg_dev_env_v2_demoable/datetime_modelling_and_ref_frames/MATLAB Function6 ==
  data: T0 input; GMST_angle output; hour input; min input; sec input
function GMST_angle = calc_GMST_angle_from_T0(T0, hour, min, sec)

% calculates GMST_angle in units of seconds (longitudinal seconds)
GMST_angle = 24110.54841 + 8640184.812866 * T0 + 0.093104 * T0^2 ...
    - 6.2e-6 * T0^3 + 1.002737909350795 * (3600*hour + 60*min + sec);

% reduces to range of 0-86400
GMST_angle = mod(GMST_angle, 86400);

% converts to degrees (there are 240 longitudinal seconds in a degree)
GMST_angle = GMST_angle / 240;

== matlab function cubesat_alg_dev_env_v2_demoable/datetime_modelling_and_ref_frames/MATLAB Function7 ==
  data: GMST_angle input; GCI_to_ECEF output
function GCI_to_ECEF = calc_GCI_to_ECEF_from_GMST_angle(GMST_angle)

% calculates the transformation matrix from GCI to ECEF
GCI_to_ECEF = [cos(GMST_angle) sin(GMST_angle) 0 ; ...
    -sin(GMST_angle) cos(GMST_angle) 0 ; 0 0 1];

== matlab function cubesat_alg_dev_env_v2_demoable/datetime_modelling_and_ref_frames/MATLAB Function8 ==
  data: pos input; geodetic_lat output; a input; b input; geodetic_long output; geodetic_height output
function [geodetic_lat, geodetic_long, geodetic_height] = ...
    ECEF_coords_to_geodetic(pos, a, b)

    % converts from ECEF coordinates to geodetic coordinates

    x = pos(1);
    y = pos(2);
    z = pos(3);

    e2 = 1 - b^2 / a^2;
    eps2 = a^2 / b^2 - 1;
    rho = sqrt(x^2 + y^2);

    p = abs(z)/eps2;
    s = rho^2/(e2*eps2);
    q = p^2 - b^2 + s;

    u = p/sqrt(q);
    v = b^2*u^2/q;
    P=27*v*s/q;
    Q=(sqrt(P+1) + sqrt(P))^(2/3);

    t=(1+Q+1/Q)/6;
    c=sqrt(u^2-1+2*t);
    w=(c-u)/2;

    d=sign(z)*sqrt(q)*(w+sqrt(t^2+v)-u*w-t/2-1/4);

    N = a*sqrt(1+eps2*d^2/b^2);
    lat = asin((eps2+1)*(d/N));
    
    h = rho*cos(lat)+z*sin(lat)-a^2/N;
    long = atan2(y, x);

    % converts from rad to deg
    geodetic_lat = rad2deg(lat);
    geodetic_long = rad2deg(long);

    geodetic_height = h;

== matlab function cubesat_alg_dev_env_v2_demoable/attitude_determination_and_vehicle_est/MATLAB Function5 ==
  data: u input; y output
function y = noise_sim(u)

y = u;

== matlab function cubesat_alg_dev_env_v2_demoable/attitude_determination_and_vehicle_est/Creates UV Values ==
  data: r_sat_com input; st1 output; r_sat_com_ax1 input; r_sat_com_ax2 input; q_sat_com input; st2 output
function [st1,st2] = fcn(r_sat_com,r_sat_com_ax1,r_sat_com_ax2,q_sat_com)
st1 = 0;
st2 = 0;

q_sat_com_reshape = reshape(q_sat_com,[1 4]);
r_sat_com_reshape = reshape(r_sat_com, [1 3]);

r_ref_com = quatrotate(q_sat_com_reshape,r_sat_com_reshape);

st1 = dot(r_ref_com,r_sat_com_ax1);
st2 = dot(r_ref_com,r_sat_com_ax2);

end

function v2 = quatrotate(q,v)
q0 = q(1);
q1 = q(2);
q2 = q(3);
q3 = q(4);

M = zeros(3);

M(1,1) = 1 - 2*q2^2 - 2*q3^2;
M(1,2) = 2*(q1*q2 + q0*q3);
M(1,3) = 2*(q1*q3-q0*q2);
M(2,1) = 2*(q1*q2-q0*q3);
M(2,2) = 1 - 2*q1^2 - 2*q3^2;
M(2,3) = 2*(q2*q3+q0*q1);
M(3,1) = 2*(q1*q3+q0*q2);
M(3,2) = 2*(q2*q3-q0*q1);
M(3,3) = 1 - 2*q2^2 - 2*q3^2;


v2 = (M*(v'))';
end

== matlab function cubesat_alg_dev_env_v2_demoable/attitude_determination_and_vehicle_est/Regenerates from UV Values ==
  data: r_sat_com input; r_ref_com_est output; r_sat_com_ax1 input; r_sat_com_ax2 input; st1 input; st2 input
function r_ref_com_est = fcn(r_sat_com,r_sat_com_ax1,r_sat_com_ax2,st1,st2)

r_ref_com_est_unshaped =   r_sat_com_ax1*st1 + r_sat_com_ax2*st2 ...
                + r_sat_com*sqrt(1-st1^2-st2^2);

r_ref_com_est = reshape(r_ref_com_est_unshaped,[1 3]);

== matlab function cubesat_alg_dev_env_v2_demoable/attitude_determination_and_vehicle_est/MATLAB Function1 ==
  data: u input; y output
function y = noise_sim(u)
y = u;
end

== matlab function cubesat_alg_dev_env_v2_demoable/attitude_determination_and_vehicle_est/MEKF ==
  data: P input; P output; q_n2m input; beta input; q_n2m output; beta output; omega input; ref_ss input; mes_ss input; use_sun_sensor input; ref_mag input; mes_mag input; use_magnometer input; ref_aam input; mes_aam input; use_ang_acc_magentorquer input; use_ang_vel input; mes_var_ss input; mes_var_mg input; mes_var_aam input; dt input; hat_omega output size=[3,1]; use_steve_mode input; steve_ref input; steve_mes input
function [P, q_n2m,beta,hat_omega] = fcn(P,q_n2m,beta,omega, ref_ss, mes_ss, use_sun_sensor, ref_mag, mes_mag, ...
                                            use_magnometer, ref_aam, mes_aam, use_ang_acc_magentorquer, use_ang_vel, mes_var_ss, mes_var_mg, mes_var_aam, dt, use_steve_mode, steve_ref, steve_mes)
    delta_x = zeros(6,1);

    G = [-eye(3), zeros(3);
    zeros(3), eye(3)];

    Q = [mes_var_ss^2*eye(3), zeros(3);
    zeros(3), mes_var_mg^2*eye(3)];

    %sun sensor
    if use_sun_sensor
    [q_n2m,P,delta_x] = mekf(mes_ss,ref_ss,P,mes_var_ss,q_n2m,delta_x);
    end

    %magnometer
    if use_magnometer
    [q_n2m,P,delta_x] = mekf(mes_mag,ref_mag,P,mes_var_mg,q_n2m,delta_x);
    end

    %steve mode
    if use_steve_mode 
        steve_mes_reshape = reshape(steve_mes,[1 3]);
        steve_ref_reshape = reshape(steve_ref,[1 3]);
        [q_n2m,P,delta_x] = mekf(steve_mes_reshape,steve_ref_reshape,P,0.1,q_n2m,delta_x);
    end
    
    %angular velocity with accelerometer
    %if use_ang_acc_magentorquer
    %[q_n2m,P,delta_x] = mekf(mes_aam,ref_aam,P,mes_var_aam,q_n2m,delta_x);
    %end


    x_extra = [0 ; delta_x(1:3)]';

    q_n2m = q_n2m + (0.5*quatmultiply(q_n2m,x_extra));
    q_n2m = q_n2m/norm(q_n2m);

    hat_omega = zeros(3,1);
    if use_ang_vel
        %beta = beta + delta_x(4:6);
        hat_omega(1) = omega(1) - beta(1);
        hat_omega(2) = omega(2) - beta(2);
        hat_omega(3) = omega(3) - beta(3);
    end

    x_extra = [0; hat_omega]';
    dot_q_n2m = 0.5*quatmultiply(q_n2m,x_extra);

    q_n2m = q_n2m + dot_q_n2m*dt;
    q_n2m = q_n2m/norm(q_n2m);

    w = [ 0  -hat_omega(3),  hat_omega(2);
          hat_omega(3),    0, -hat_omega(1);
         -hat_omega(2),  hat_omega(1),    0];
    
    F = [-w, eye(3);
        zeros(3), zeros(3)];

    dot_P = F*P + P*F'+G*Q*G';

    P = P + dot_P*dt;

end


function [q_n2m,P,delta_x] = mekf(b,r,P,R,q_n2m, delta_x)

    b_est = quatrotate(q_n2m,r);
    b01 = b_est(1);
    b02 = b_est(2);
    b03 = b_est(3);
    
    
    H = [   0  -b03,  b02,  0,  0,  0;
          b03,    0, -b01,  0,  0,  0;
         -b02,  b01,    0,  0,  0,  0];
    
    K = P*transpose(H)/(H*P*transpose(H)+R^2*eye(3));
    
    epsilon = (b - quatrotate(q_n2m,r));
    
    delta_x = delta_x + K*(epsilon'-H*delta_x);
    
    P = (eye(6) - K*H)*P;

end

function v = quatrotate(q,v)
q0 = q(1);
q1 = q(2);
q2 = q(3);
q3 = q(4);

M = zeros(3);

M(1,1) = 1 - 2*q2^2 - 2*q3^2;
M(1,2) = 2*(q1*q2 + q0*q3);
M(1,3) = 2*(q1*q3-q0*q2);
M(2,1) = 2*(q1*q2-q0*q3);
M(2,2) = 1 - 2*q1^2 - 2*q3^2;
M(2,3) = 2*(q2*q3+q0*q1);
M(3,1) = 2*(q1*q3+q0*q2);
M(3,2) = 2*(q2*q3-q0*q1);
M(3,3) = 1 - 2*q2^2 - 2*q3^2;

v = (M*(v'))';
end

== matlab function cubesat_alg_dev_env_v2_demoable/attitude_determination_and_vehicle_est/MATLAB Function2 ==
  data: u input; y output
function y = noise_sim(u)

y = u;

== matlab function cubesat_alg_dev_env_v2_demoable/env_modelling/MATLAB Function ==
  data: pos_gci input; torque_body output; iner_tensor input
function torque_body  = grav_grad_torque(pos_gci, iner_tensor)
    % mass of earth, grav constant
    m_e = 5.97219e24;
    G = 6.67430e-11;

    % grav param
    u = G*m_e;

    radius = norm(pos_gci);
    nadir_vec = -normalize(pos_gci);
    torque_body = cross(3*u/radius^3*nadir_vec, ...
        iner_tensor*nadir_vec);

== matlab function cubesat_alg_dev_env_v2_demoable/attitude_determination_and_vehicle_est/MATLAB Function3 ==
  data: u input; y output
function y = noise_sim(u)

y = u';

== matlab function cubesat_alg_dev_env_v2_demoable/datetime_modelling_and_ref_frames/MATLAB Function1 ==
  data: datetime input; dyear output
function dyear = dyear_from_datetime(datetime)

    % the datetime format is provided as a 6 value array
    % year, month, day, hour, minute, second

    % sequentially builds the decimal year

    % potentially we may want to use /61 for leap second days but this is
    % likely fine as our simulation just needs to perform regular datetime
    % updates for simple testing

    tot_mins = datetime(5) + datetime(6) / 60;
    tot_hours = datetime(4) + tot_mins / 60;
    tot_days = datetime(3) + tot_hours / 24;
    tot_months = datetime(2) + tot_days / (275/9); % average days in month across year
    tot_years = datetime(1) + tot_months / 12;

    dyear = tot_years;

== matlab function cubesat_alg_dev_env_v2_demoable/attitude_determination_and_vehicle_est/MATLAB Function4 ==
  data: u input; y output
function y = signal_cleanup(u)
y = [0,0,0];

if u(1) == 0
    y(1) = -u(2);
else
    y(1) = u(1);
end

if u(3) == 0
    y(2) = -u(4);
else
    y(2) = u(3);
end

if u(5) == 0
    y(3) = -u(6);
else
    y(3) = u(5);
end


end
